simulink model "part2_2017b"  (R2017b)
settings: Solver=FixedStepAuto  StartTime=0.0  StopTime=500  FixedStep=0.1  RelTol=1e-3
values from neighbouring files (symbols this model uses):
  thrusters =     [thrusters.mat]
undefined symbols (not defined in the file or in its folder): Hoerner, vessel
libraries: marine_hydro x2, marine_gnc x1
settings Model: Creator=jonbjor  LastModifiedBy=jonbjor

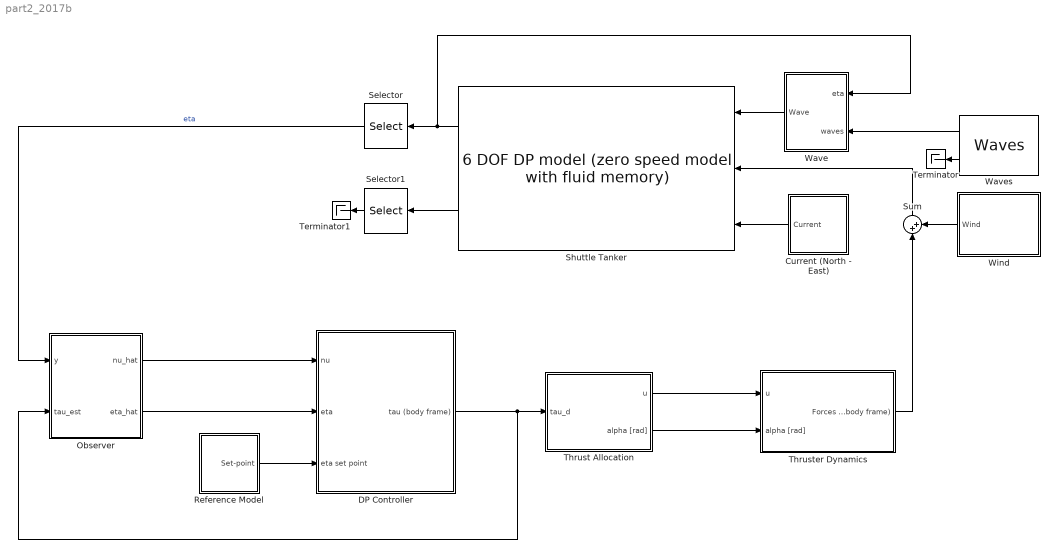
== system part2_2017b ==
  Current (North - East) : Subsystem
  DP Controller : Subsystem
  Observer : Subsystem
  Reference Model : Subsystem
  Selector : Selector  InputPortWidth=6  IndexOptions=Index vector (dialog)  Indices=[1 2 6]  OutputSizes=1
  Selector1 : Selector  InputPortWidth=6  IndexOptions=Index vector (dialog)  Indices=[1 2 6]  OutputSizes=1
  Shuttle Tanker : marine_hydro/Hydro Library/6 DOF DP model  (zero speed model with fluid memory)  ABC=vesselABC  rho=1025  Axc=0.9*vessel.main.T*vessel.main.B  Ayc=0.9*vessel.main.T*vessel.main.Lpp  CX=1  CY_2D=Hoerner(vessel.main.B,vessel.main.T)  Bv=vessel.Bv  mask(6 DOF zero speed model){}
      link override "Integrator1 ": InitialCondition=nu0
      link override Integrator2: InitialCondition=eta0
      settings: SourceProductName=MSS Hydro
      mask Display:
      | image('shuttleTanker.jpg');
      | color('white'); port_label('output', 1, 'eta')
      | color('white'); port_label('output', 2, 'nu')
      | color('white'); port_label('input', 1, 'tau_wave')
      | color('white'); port_label('input', 2, 'tau')
      | color('white'); port_label('input', 3, 'nu_c')
  Sum : Sum  Inputs=|++
  Terminator : Terminator
  Terminator1 : Terminator
  Thrust Allocation : Subsystem
  Thruster Dynamics : Subsystem  mask{thrusterfault=off}
      mask prompts: thrusterfault "Fault on thruster #2 and #5?"
  Wave : Subsystem  mask{waveforces=on}
      mask prompts: waveforces "Waveforces enabled"
  Waves : marine_gnc/Environment/Waves/Waves  spectrum_type=ITTC  disp_flag=on  plot_spectrum=off  plot_realization=off  hs=5  omega_peak=pi/10  psi_mean=0  gamma=-1  spread=2  depth=inf  nfreq=20  ndir=10  energylim=0.005  freq_cutoff=3  dir_cutoff=0  rand_seed=123  rand_freq=on  rand_dir=on  Zeta_a=0  Omega=0  Phase=0  Wavenum=0  Psi=0
      settings: SourceProductName=MSS GNC
  Wind : Subsystem
  wires:
  Shuttle Tanker/2 -> Selector1/1
  Reference Model/1(Set-point) -> DP Controller/3(eta set point)
  DP Controller/1(tau (body frame)) -> Thrust Allocation/1(tau_d), Observer/2(tau_est)
  Shuttle Tanker/1 -> Wave/1(eta), Selector/1
  Current (North - East)/1(Current) -> Shuttle Tanker/3
  Wave/1(Wave) -> Shuttle Tanker/1
  Waves/1 -> Wave/2(waves)
  Waves/2 -> Terminator/1
  Selector1/1 -> Terminator1/1
  Observer/2(eta_hat) -> DP Controller/2(eta)
  Observer/1(nu_hat) -> DP Controller/1(nu)
  Thrust Allocation/1(u) -> Thruster Dynamics/1(u)
  Wind/1(Wind) -> Sum/2
  Thruster Dynamics/1("Forces (body frame) ") -> Sum/1
  Sum/1 -> Shuttle Tanker/2
  Thrust Allocation/2(alpha [rad]) -> Thruster Dynamics/2(alpha [rad])
  Selector/1 -> Observer/1(y)  "eta"

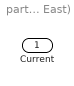
== system part2_2017b/Current (North - East) ==
  Current : Outport

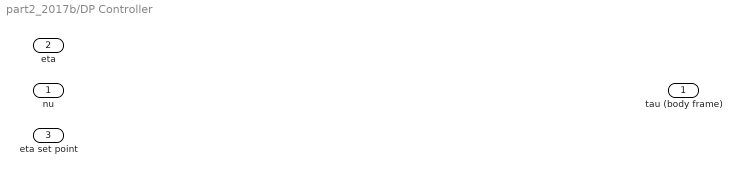
== system part2_2017b/DP Controller ==
  nu : Inport
  eta : Inport  Port=2
  eta set point : Inport  Port=3
  tau (body frame) : Outport

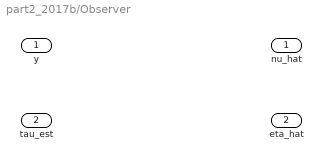
== system part2_2017b/Observer ==
  y : Inport
  tau_est : Inport  Port=2
  nu_hat : Outport
  eta_hat : Outport  Port=2

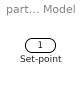
== system part2_2017b/Reference Model ==
  Set-point : Outport

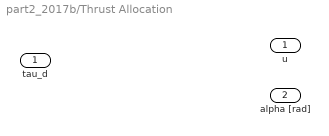
== system part2_2017b/Thrust Allocation ==
  tau_d : Inport
  u : Outport
  alpha [rad] : Outport  Port=2

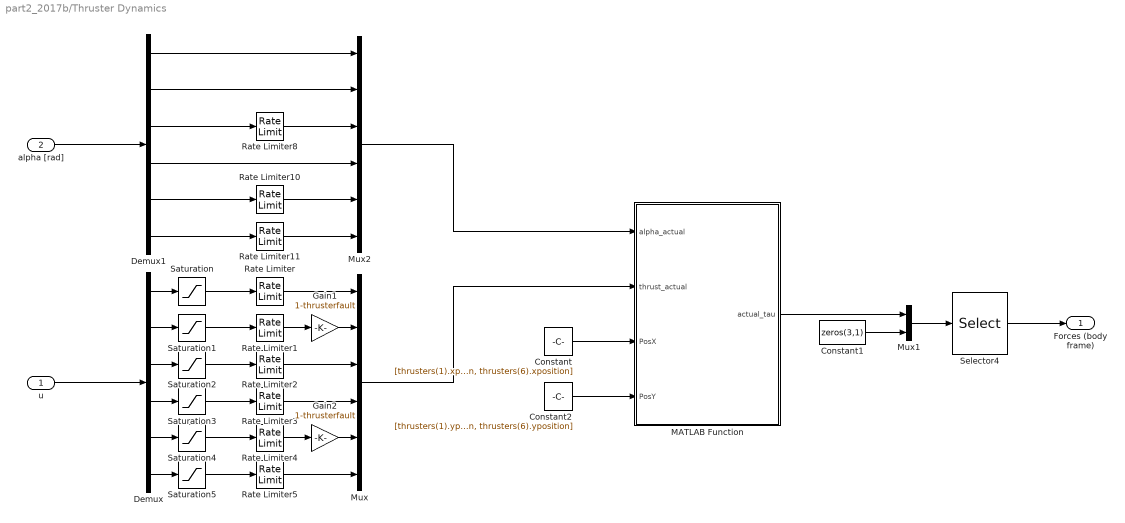
== system part2_2017b/Thruster Dynamics ==
  u : Inport
  alpha [rad] : Inport  Port=2
  Constant : Constant  Value=[thrusters(1).xposition, thrusters(2).xposition, thrusters(3).xposition, thrusters(4).xposition, thrusters(5).xposition, thrusters(6).xposition]
  Constant1 : Constant  Value=zeros(3,1)
  Constant2 : Constant  Value=[thrusters(1).yposition, thrusters(2).yposition, thrusters(3).yposition, thrusters(4).yposition, thrusters(5).yposition, thrusters(6).yposition]
  Demux : Demux  Outputs=6
  Demux1 : Demux  Outputs=6
  Gain1 : Gain  Gain=1-thrusterfault
  Gain2 : Gain  Gain=1-thrusterfault
  MATLAB Function : MATLAB Function  TreatAsAtomicUnit=on
  Mux : Mux  Inputs=6
  Mux1 : Mux  Inputs=2
  Mux2 : Mux  Inputs=6
  Rate Limiter : RateLimiter  RisingSlewLimit=thrusters(1).rate  FallingSlewLimit=-thrusters(1).rate  SampleTimeMode=inherited
  Rate Limiter1 : RateLimiter  RisingSlewLimit=thrusters(2).rate  FallingSlewLimit=-thrusters(2).rate  SampleTimeMode=inherited
  Rate Limiter10 : RateLimiter  RisingSlewLimit=thrusters(5).rotationspeed  FallingSlewLimit=-thrusters(5).rotationspeed  SampleTimeMode=inherited
  Rate Limiter11 : RateLimiter  RisingSlewLimit=thrusters(6).rotationspeed  FallingSlewLimit=-thrusters(6).rotationspeed  SampleTimeMode=inherited
  Rate Limiter2 : RateLimiter  RisingSlewLimit=thrusters(3).rate  FallingSlewLimit=-thrusters(3).rate  SampleTimeMode=inherited
  Rate Limiter3 : RateLimiter  RisingSlewLimit=thrusters(4).rate  FallingSlewLimit=-thrusters(4).rate  SampleTimeMode=inherited
  Rate Limiter4 : RateLimiter  RisingSlewLimit=thrusters(5).rate  FallingSlewLimit=-thrusters(5).rate  SampleTimeMode=inherited
  Rate Limiter5 : RateLimiter  RisingSlewLimit=thrusters(6).rate  FallingSlewLimit=-thrusters(6).rate  SampleTimeMode=inherited
  Rate Limiter8 : RateLimiter  RisingSlewLimit=thrusters(3).rotationspeed  FallingSlewLimit=-thrusters(3).rotationspeed  SampleTimeMode=inherited
  Saturation : Saturate  UpperLimit=thrusters(1).thrust  LowerLimit=-thrusters(1).thrust
  Saturation1 : Saturate  UpperLimit=thrusters(2).thrust  LowerLimit=-thrusters(2).thrust
  Saturation2 : Saturate  UpperLimit=thrusters(3).thrust  LowerLimit=-thrusters(3).thrust
  Saturation3 : Saturate  UpperLimit=thrusters(4).thrust  LowerLimit=-thrusters(4).thrust
  Saturation4 : Saturate  UpperLimit=thrusters(5).thrust  LowerLimit=-thrusters(5).thrust
  Saturation5 : Saturate  UpperLimit=thrusters(6).thrust  LowerLimit=-thrusters(6).thrust
  Selector4 : Selector  InputPortWidth=6  IndexOptions=Index vector (dialog)  Indices=[1 2 4 5 6 3]  OutputSizes=1
  "Forces (body frame) " : Outport
  wires:
  Rate Limiter2/1 -> Mux/3
  Saturation/1 -> Rate Limiter/1
  Mux1/1 -> Selector4/1
  Constant1/1 -> Mux1/2
  Demux/5 -> Saturation4/1
  Demux/4 -> Saturation3/1
  Saturation4/1 -> Rate Limiter4/1
  Demux/2 -> Saturation1/1
  Saturation1/1 -> Rate Limiter1/1
  Demux/1 -> Saturation/1
  Demux/3 -> Saturation2/1
  Saturation2/1 -> Rate Limiter2/1
  Saturation3/1 -> Rate Limiter3/1
  Selector4/1 -> "Forces (body frame) "/1
  Gain1/1 -> Mux/2
  Rate Limiter3/1 -> Mux/4
  Rate Limiter1/1 -> Gain1/1
  Rate Limiter/1 -> Mux/1
  Rate Limiter4/1 -> Gain2/1
  Saturation5/1 -> Rate Limiter5/1
  Demux/6 -> Saturation5/1
  Rate Limiter5/1 -> Mux/6
  Gain2/1 -> Mux/5
  Demux1/6 -> Rate Limiter11/1
  Demux1/3 -> Rate Limiter8/1
  Rate Limiter11/1 -> Mux2/6
  Rate Limiter10/1 -> Mux2/5
  Demux1/2 -> Mux2/2
  Demux1/1 -> Mux2/1
  Demux1/4 -> Mux2/4
  Rate Limiter8/1 -> Mux2/3
  Demux1/5 -> Rate Limiter10/1
  u/1 -> Demux/1
  alpha [rad]/1 -> Demux1/1
  Constant/1 -> MATLAB Function/3(PosX)
  Constant2/1 -> MATLAB Function/4(PosY)
  Mux/1 -> MATLAB Function/2(thrust_actual)
  Mux2/1 -> MATLAB Function/1(alpha_actual)
  MATLAB Function/1(actual_tau) -> Mux1/1

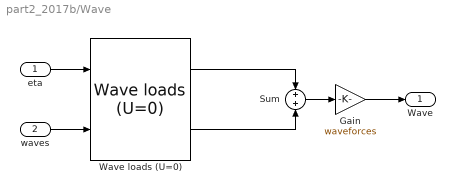
== system part2_2017b/Wave ==
  eta : Inport
  waves : Inport  Port=2
  Gain : Gain  Gain=waveforces
  Sum : Sum
  Wave loads (U=0) : marine_hydro/Hydro Library/Wave loads (U=0)
      settings: SourceProductName=MSS Hydro
  Wave : Outport
  wires:
  eta/1 -> Wave loads (U=0)/1
  waves/1 -> Wave loads (U=0)/2
  Sum/1 -> Gain/1
  Wave loads (U=0)/1 -> Sum/1
  Wave loads (U=0)/2 -> Sum/2
  Gain/1 -> Wave/1

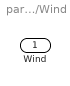
== system part2_2017b/Wind ==
  Wind : Outport

== matlab function part2_2017b/Thruster Dynamics/MATLAB Function ==
  data: alpha_actual input; thrust_actual input; actual_tau output; PosX input; PosY input
function actual_tau   = fcn(alpha_actual,thrust_actual,PosX,PosY)

    Alpha_surge =[cos(alpha_actual(1)) cos(alpha_actual(2)) cos(alpha_actual(3)) cos(alpha_actual(4)) cos(alpha_actual(5)) cos(alpha_actual(6))];  
    Alpha_sway = [sin(alpha_actual(1)) sin(alpha_actual(2)) sin(alpha_actual(3)) sin(alpha_actual(4)) sin(alpha_actual(5)) sin(alpha_actual(6))];
    Alpha_yaw = [sin(alpha_actual(1))*PosX(1)-cos(alpha_actual(1))*PosY(1) sin(alpha_actual(2))*PosX(2)-cos(alpha_actual(2))*PosY(2) ...
                 sin(alpha_actual(3))*PosX(3)-cos(alpha_actual(3))*PosY(3) sin(alpha_actual(4))*PosX(4)-cos(alpha_actual(4))*PosY(4) ...
                 sin(alpha_actual(5))*PosX(5)-cos(alpha_actual(5))*PosY(5) sin(alpha_actual(6))*PosX(6)-cos(alpha_actual(6))*PosY(6)];

    actual_tau = [Alpha_surge; Alpha_sway; Alpha_yaw]*thrust_actual;
end
